simulink model "main2"  (Simulink 7.3)
settings: Solver=ode45  StartTime=0.0  StopTime=10.0  RelTol=1e-8
libraries: simulink x1
settings Model: Creator=Sain  LastModifiedBy=Sain

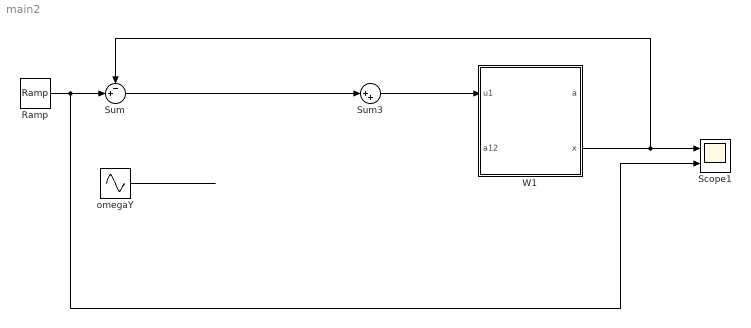
== system main2 ==
  Ramp : simulink/Sources/Ramp  SystemSampleTime=-1  slope=60  start=0  X0=0
  Scope1 : Scope  NumInputPorts=2
      settings: YMin=-5~-5  YMax=5~5
  Sum : Sum  Inputs=-+|  OutDataType=fixdt(1, 16)  OutScaling=2^0
  Sum3 : Sum  Inputs=|++  OutDataType=fixdt(1, 16)  OutScaling=2^0
  W1 : Subsystem
  omegaY : Sin  Amplitude=1  Bias=0  Frequency=2  Phase=0  Samples=10  SampleTime=0  Offset=0
  wires:
  Sum3/1 -> W1/1(u1)
  omegaY/1 -> ?
  Ramp/1 -> Sum/2, Scope1/2
  W1/2(x) -> Sum/1, Scope1/1
  Sum/1 -> Sum3/1

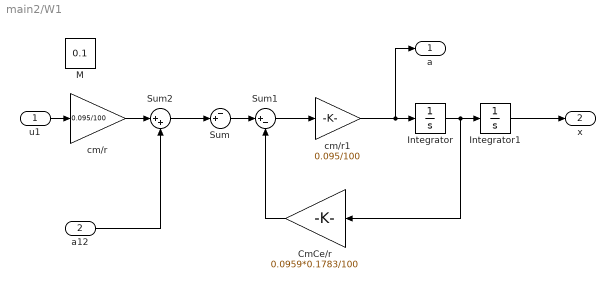
== system main2/W1 ==
  u1 : Inport  OutDataType=fixdt(1, 16)  OutScaling=2^0
  a12 : Inport  Port=2  OutDataType=fixdt(1, 16)  OutScaling=2^0
  CmCe/r : Gain  Gain=0.0959*0.1783/100  ParameterDataType=fixdt(1, 16)  ParameterScaling=2^0  OutDataType=fixdt(1, 16)  OutScaling=2^0
  Integrator : Integrator
  Integrator1 : Integrator
  M : Constant  Value=0.1  OutDataType=fixdt(1, 16)  OutScaling=2^0
  Sum : Sum  Inputs=-+|  OutDataType=fixdt(1, 16)  OutScaling=2^0
  Sum1 : Sum  Inputs=|+-  OutDataType=fixdt(1, 16)  OutScaling=2^0
  Sum2 : Sum  Inputs=|++  OutDataType=fixdt(1, 16)  OutScaling=2^0
  cm/r : Gain  Gain=0.095/100  ParameterDataType=fixdt(1, 16)  ParameterScaling=2^0  OutDataType=fixdt(1, 16)  OutScaling=2^0
  cm/r1 : Gain  Gain=0.095/100  ParameterDataType=fixdt(1, 16)  ParameterScaling=2^0  OutDataType=fixdt(1, 16)  OutScaling=2^0
  a : Outport  OutDataType=fixdt(1, 16)  OutScaling=2^0
  x : Outport  Port=2  OutDataType=fixdt(1, 16)  OutScaling=2^0
  wires:
  u1/1 -> cm/r/1
  Integrator/1 -> Integrator1/1, CmCe/r/1
  Integrator1/1 -> x/1
  cm/r/1 -> Sum2/1
  a12/1 -> Sum2/2
  Sum1/1 -> cm/r1/1
  Sum2/1 -> Sum/2
  Sum/1 -> Sum1/1
  CmCe/r/1 -> Sum1/2
  cm/r1/1 -> Integrator/1, a/1
